simulink model "Task2_motor_speed"  (R2021b)
settings: Solver=VariableStepAuto  StartTime=0.0  StopTime=10.0  RelTol=1e-3
values from neighbouring files (symbols this model uses):
  b = 0.1    [task_motor_speed_input.m]
  J = 0.01    [task_motor_speed_input.m]
  K = 0.01    [task_motor_speed_input.m]
  L = 0.5    [task_motor_speed_input.m]
  R = 1    [task_motor_speed_input.m]
  v = 12    [task_motor_speed_input.m]
settings Model: Creator=vinod  LastModifiedBy=vinod

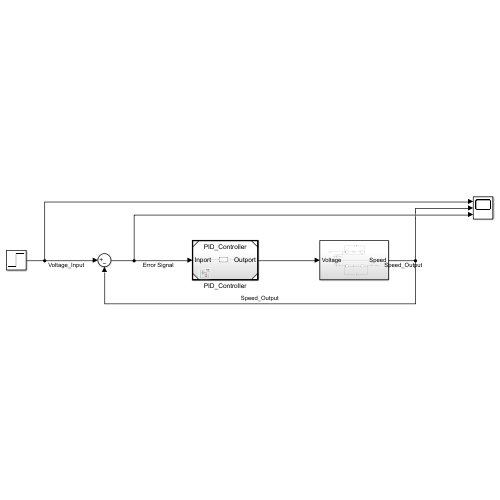
[thumbnail: Simulink's stored preview of the top-level diagram]
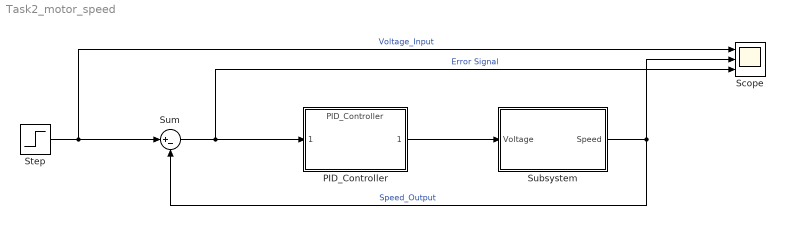
== system Task2_motor_speed ==
  PID_Controller : ModelReference  ModelNameDialog=PID_Controller  SimulationMode=Normal  ModelReferenceVersion=1.10
  Scope : Scope  NumInputPorts=3
  Step : Step  Time=0  After=v  SampleTime=0.01
  Subsystem : Subsystem
  Sum : Sum  Inputs=|+-
  wires:
  PID_Controller/1 -> Subsystem/1(Voltage)
  Subsystem/1(Speed) -> Scope/2, Sum/2  "Speed_Output"
  Sum/1 -> Scope/3, PID_Controller/1  "Error Signal"
  Step/1 -> Scope/1, Sum/1  "Voltage_Input"

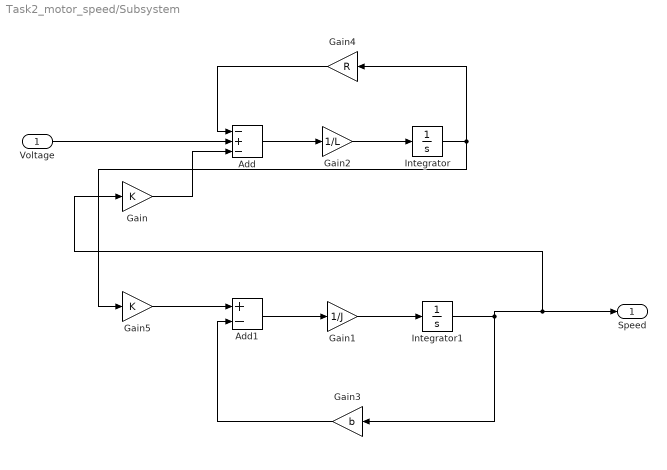
== system Task2_motor_speed/Subsystem ==
  Voltage : Inport
  Add : Sum  Inputs=-+-
  Add1 : Sum  Inputs=+-
  Gain : Gain  Gain=K
  Gain1 : Gain  Gain=1/J
  Gain2 : Gain  Gain=1/L
  Gain3 : Gain  Gain=b
  Gain4 : Gain  Gain=R
  Gain5 : Gain  Gain=K
  Integrator : Integrator
  Integrator1 : Integrator
  Speed : Outport
  wires:
  Integrator1/1 -> Speed/1, Gain/1, Gain3/1
  Gain1/1 -> Integrator1/1
  Gain/1 -> Add/3
  Add1/1 -> Gain1/1
  Integrator/1 -> Gain4/1, Gain5/1
  Voltage/1 -> Add/2
  Gain5/1 -> Add1/1
  Gain4/1 -> Add/1
  Add/1 -> Gain2/1
  Gain2/1 -> Integrator/1
  Gain3/1 -> Add1/2
